simulink model "mech_fceng"  (Simulink 6.0)
settings: Solver=ode45  StartTime=0.0  StopTime=inf  RelTol=1e-3  AbsTol=1e-4
PreLoadFcn:
  | mech_fceng_init;load mech_fceng_images;
InitFcn:
  | mech_slider_open(gcs);
values from neighbouring files (symbols this model uses):
  Cv = 2000    [mech_transmission_data.mat]
  G = 9.81    [mech_motorcycle_data.m]
  m = 161    [mech_transmission_data.mat]
  N = 270    [mech_transmission_data.mat]
  R = 1    [clutchparam.mat]    (also in mech_toroid_setup.m = 10; mech_transmission_data.mat = 5)
undefined symbols (not defined in the file or in its folder): AirRo, Pa, Q, Ta, Vo, Vtdc
libraries: mblibv1 x47, simulink x3, simulink_extras x1
(part 1 of 2)
settings Model: Creator=arnav  LastModifiedBy=batserve  ExtModeAutoUpdateStatusClock=off  ProdHWDeviceType=Specified
settings DataIOCC: SignalLoggingName=sigsOut
settings OptimizationCC: BooleanDataType=off
settings DebuggingCC: CheckExecutionContextPreStartOutputMsg=on  CheckExecutionContextRuntimeOutputMsg=on  SolverPrmCheckMsg=none  UnconnectedInputMsg=none  UnconnectedOutputMsg=none  UnconnectedLineMsg=none
settings HardwareCC: ProdHWDeviceType=Specified
settings SimMechanicsCC: WarnOnRedundantConstraints=off

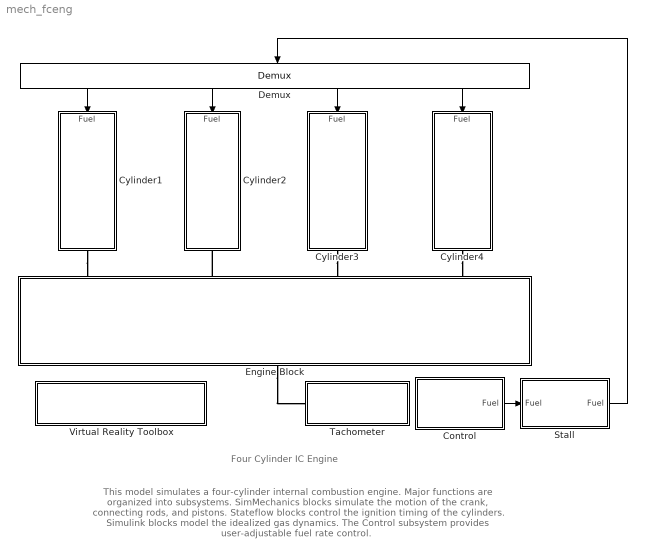
== system mech_fceng ==
  note: This model simulates a four-cylinder internal combustion engine. Major functions are organized into subsystems.
      | SimMechanics blocks simulate the motion of the crank, connecting rods, and pistons. Stateflow blocks
      | control the ignition timing of the cylinders. Simulink blocks model the idealized gas dynamics. The Control
      | subsystem provides user-adjustable fuel rate control.
  note: Four Cylinder IC Engine
  Control : Subsystem  Tag=OpenMeAtStartUp
  Cylinder1 : Subsystem  Orientation=down
      mask Display: image(crodassm);
  Cylinder2 : Subsystem  Orientation=down
      mask Display: image(crodassmb);
  Cylinder3 : Subsystem  Orientation=down
      mask Display: image(crodassmb);
  Cylinder4 : Subsystem  Orientation=down
      mask Display: image(crodassm);
  Demux : Demux  Orientation=down
  Engine Block : Subsystem  Orientation=up
      mask Display: image(crank);
  Stall : Subsystem
  Tachometer : Subsystem
  Virtual Reality Toolbox : Subsystem
      settings: OpenFcn=mech_OpenVrWorld(gcs,'mech_fceng_vrlib')
      mask Type: Double-click open
      mask Display: disp(sprintf('Double-click to open\nVirtual Reality Toolbox viewer'))
  wires:
  Demux/1 -> Cylinder1/1(Fuel)
  Demux/2 -> Cylinder2/1(Fuel)
  Demux/3 -> Cylinder3/1(Fuel)
  Demux/4 -> Cylinder4/1(Fuel)
  Control/1(Fuel) -> Stall/1("Fuel ")
  Stall/1(Fuel) -> Demux/1
  connections:
  Cylinder1/RConn1 -- Engine Block/RConn1
  Cylinder4/RConn1 -- Engine Block/RConn4
  Engine Block/LConn1 -- Tachometer/LConn1
  Cylinder3/RConn1 -- Engine Block/RConn3
  Engine Block/RConn2 -- Cylinder2/RConn1

== system mech_fceng/Control ==
  Constant : Constant
  Cylinder1 : simulink/Signal Routing/Manual Switch  Orientation=down  sw=0  action=0
  Cylinder4 : simulink/Signal Routing/Manual Switch  Orientation=down  sw=0  action=0
  Fuel Control : simulink/Math Operations/Slider Gain  Tag="674   438   332   100"  low=0  gain=2  high=4
  OFF : Constant  Orientation=up  Value=0
  ON : Constant  Orientation=up  Value=-1
  Fuel : Outport
  tag scope: Cylinder1=global, Cylinder2=global
  wires:
  Cylinder1/1 -> [Cylinder1]
  Constant/1 -> Fuel Control/1
  Fuel Control/1 -> Fuel/1
  OFF/1 -> Cylinder1/1, Cylinder4/1
  ON/1 -> Cylinder4/2, Cylinder1/2
  Cylinder4/1 -> [Cylinder2]

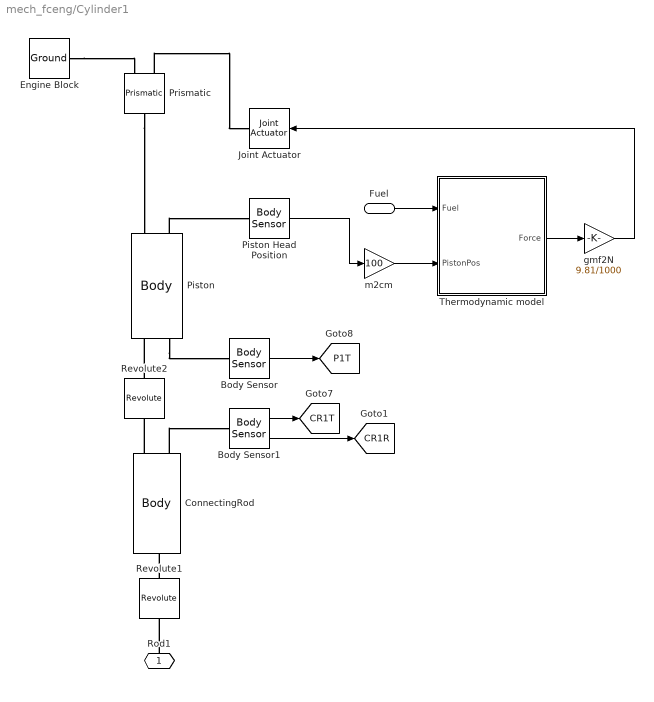
== system mech_fceng/Cylinder1 ==
  Fuel : Inport  Port=1  LatchInput=off
  Body Sensor : mblibv1/Sensors &  Actuators/Body Sensor  Opaque=on  PhysicalDomain=Mechanical  PortType=blob  Muxed=on  Pose=off  Angle=on  AngleUnits=deg  ArcVelocity=off  ArcVelocityUnits=deg/s  ArcAcceleration=off  ArcAccelerationUnits=deg/s^2  CoordPosition=on  CoordPositionUnits=m  Velocity=off  VelocityUnits=m/s  Acceleration=off  AccelerationUnits=m/s^2  Quaternion=on  QuaternionDT=off  QuaternionDDT=off  QuaternionUnits=off  OutputVector=[1]  ActiveIO=on  Width=3  DialogClass=MechanicalSensorBlock  ReferenceFrame=Absolute (World)
  Body Sensor1 : mblibv1/Sensors &  Actuators/Body Sensor  Opaque=on  PhysicalDomain=Mechanical  PortType=blob  Muxed=off  Pose=on  Angle=on  AngleUnits=deg  ArcVelocity=off  ArcVelocityUnits=deg/s  ArcAcceleration=off  ArcAccelerationUnits=deg/s^2  CoordPosition=on  CoordPositionUnits=m  Velocity=off  VelocityUnits=m/s  Acceleration=off  AccelerationUnits=m/s^2  Quaternion=on  QuaternionDT=off  QuaternionDDT=off  QuaternionUnits=off  OutputVector=[ 3 9 ]  ActiveIO=on  Width=12  DialogClass=MechanicalSensorBlock  ReferenceFrame=Absolute (World)
  ConnectingRod : mblibv1/Bodies/Body  Orientation=up  PhysicalDomain=mechanical  SubClassName=Unknown  LeftPortType=workingframe  RightPortType=workingframe  LConnTagsString=CS1  RConnTagsString=CS2|CS3  DialogClass=MechanicalBodyBlock  Mass=676.73  MassUnits=g  InertiaUnits=kg*m^2  Inertia=[37007.64 0 -0.01;0 2936.99 7181.27;-0.01 7181.27 34460.53]*1E-7  Shape=Cylinder  ShapeDims=[1 1]  ShapeUnits=m  ShapeUse=false  Density=1  DensityUnits=kg/m^3  DensityUse=false  CG=Left$CG$[-18 11.35 -2.70]$WORLD$WORLD$cm$[0 0 0]$Euler X-Y-Z$deg$WORLD$false  WorkingFrames=Left$CS1$[-18 4.24 -4.24]$WORLD$WORLD$cm$[0 0 0]$Euler X-Y-Z$deg$WORLD$true#Right$CS2$[-18 23.79 0]$WORLD$WORLD$cm$[0 0 0]$Euler X-Y-Z$deg$WORLD$true#Right$CS3$[-18 4.24 -4.24]$WORLD$WORLD$cm$[0 0 0]$Euler X-Y-Z$deg$WORLD$true
  Engine Block : mblibv1/Bodies/Ground  Opaque=on  LeftPortType=env  RightPortType=workingframe  PhysicalDomain=Mechanical  DialogClass=GroundBlock  CoordPosition=[-13.23 23.79 0]  CoordPositionUnits=cm  StateVectorMgrId=-1  MachineId=[0 0]  ShowEnvPort=off
  Joint Actuator : mblibv1/Sensors &  Actuators/Joint Actuator  Orientation=left  Opaque=on  PhysicalDomain=Mechanical  PortType=blob  ActuationStyle=Force  AngleUnits=deg  ArcVelocityUnits=deg/s  ArcAccelerationUnits=deg/s^2  CoordPositionUnits=m  VelocityUnits=m/s  AccelerationUnits=m/s^2  ForceUnits=N  TorqueUnits=N-m  ActiveIO=on  Width=1  DialogClass=MechanicalActuatorBlock  Primitive=P1  ReferenceFrame=Absolute (INERTIAL)
  Piston : mblibv1/Bodies/Body  Orientation=up  PhysicalDomain=mechanical  SubClassName=Unknown  LeftPortType=workingframe  RightPortType=workingframe  LConnTagsString=CS1|CS3  RConnTagsString=CS2|CS4  DialogClass=MechanicalBodyBlock  Mass=3490.25  MassUnits=g  InertiaUnits=kg*m^2  Inertia=[39798.30 0.06 -0.01;0.06 49173.25 -0.04;-0.01 -0.04 39108.48]*1E-7  Shape=Cylinder  ShapeDims=[1 1]  ShapeUnits=m  ShapeUse=false  Density=1  DensityUnits=kg/m^3  DensityUse=false  CG=Left$CG$[-18 24.51 0]$WORLD$WORLD$cm$[0 0 0]$Euler X-Y-Z$deg$WORLD$false  WorkingFrames=Left$CS1$[-18 23.79 0]$WORLD$WORLD$cm$[0 0 0]$Euler X-Y-Z$deg$WORLD$true#Right$CS2$[-13.23 23.79 0]$WORLD$WORLD$cm$[0 0 0]$Euler X-Y-Z$deg$WORLD$true#Left$CS3$[-18 23.79 0]$WORLD$WORLD$cm$[0 0 0]$Euler X-Y-Z$deg$WORLD$true#Right$CS4$[-18 23.79+4 0]$WORLD$WORLD$cm$[0 0 0]$Euler X-Y-Z$deg$WORLD$true
  Piston Head Position : mblibv1/Sensors &  Actuators/Body Sensor  Opaque=on  PhysicalDomain=Mechanical  PortType=blob  Muxed=on  Pose=off  Angle=on  AngleUnits=deg  ArcVelocity=off  ArcVelocityUnits=deg/s  ArcAcceleration=off  ArcAccelerationUnits=deg/s^2  CoordPosition=on  CoordPositionUnits=m  Velocity=off  VelocityUnits=m/s  Acceleration=off  AccelerationUnits=m/s^2  Quaternion=on  QuaternionDT=off  QuaternionDDT=off  QuaternionUnits=off  OutputVector=[1]  ActiveIO=on  Width=3  DialogClass=MechanicalSensorBlock  ReferenceFrame=Absolute (World)
  Prismatic : mblibv1/Joints/Prismatic  Orientation=down  PhysicalDomain=mechanical  SubClassName=Unknown  LeftPortType=blob  RightPortType=blob  LConnTagsString=__newl0|SA1  RConnTagsString=__newr0  NumSAPorts=1  CutJoint=off  MarkAsCut=off  Primitives=prismatic  PrimitiveProps=P1$WORLD$[0 1 0]$prismatic  DialogClass=JointBlock
  Revolute1 : mblibv1/Joints/Revolute  Orientation=up  PhysicalDomain=mechanical  SubClassName=Unknown  LeftPortType=blob  RightPortType=blob  LConnTagsString=__newl0  RConnTagsString=__newr0  NumSAPorts=0  CutJoint=off  MarkAsCut=off  Primitives=revolute  PrimitiveProps=R1$WORLD$[1 0 0]$revolute  DialogClass=JointBlock
  Revolute2 : mblibv1/Joints/Revolute  Orientation=up  PhysicalDomain=mechanical  SubClassName=Unknown  LeftPortType=blob  RightPortType=blob  LConnTagsString=__newl0  RConnTagsString=__newr0  NumSAPorts=0  CutJoint=on  MarkAsCut=off  Primitives=revolute  PrimitiveProps=R1$WORLD$[1 0 0]$revolute  DialogClass=JointBlock
  Thermodynamic model : Subsystem
  gmf2N : Gain  Gain=9.81/1000  SaturateOnIntegerOverflow=on
  m2cm : Gain  Gain=100  SaturateOnIntegerOverflow=on
  Rod1 : PMIOPort  Orientation=up  Port=1  Side=Right
  tag scope: CR1R=global, CR1T=global, P1T=global
  wires:
  Body Sensor1/2 -> [CR1R]
  Body Sensor1/1 -> [CR1T]
  Body Sensor/1 -> [P1T]
  gmf2N/1 -> Joint Actuator/1
  Fuel/1 -> Thermodynamic model/1(Fuel)
  Piston Head Position/1 -> m2cm/1
  Thermodynamic model/1(Force) -> gmf2N/1
  m2cm/1 -> Thermodynamic model/2(PistonPos)
  connections:
  Prismatic/LConn2 -- Joint Actuator/RConn1
  Prismatic/RConn1 -- Piston/RConn1
  Engine Block/RConn1 -- Prismatic/LConn1
  ConnectingRod/RConn2 -- Body Sensor1/LConn1
  Piston/LConn2 -- Body Sensor/LConn1
  Piston/RConn2 -- Piston Head Position/LConn1
  Rod1/RConn1 -- Revolute1/LConn1
  Revolute2/RConn1 -- Piston/LConn1
  ConnectingRod/RConn1 -- Revolute2/LConn1
  Revolute1/RConn1 -- ConnectingRod/LConn1

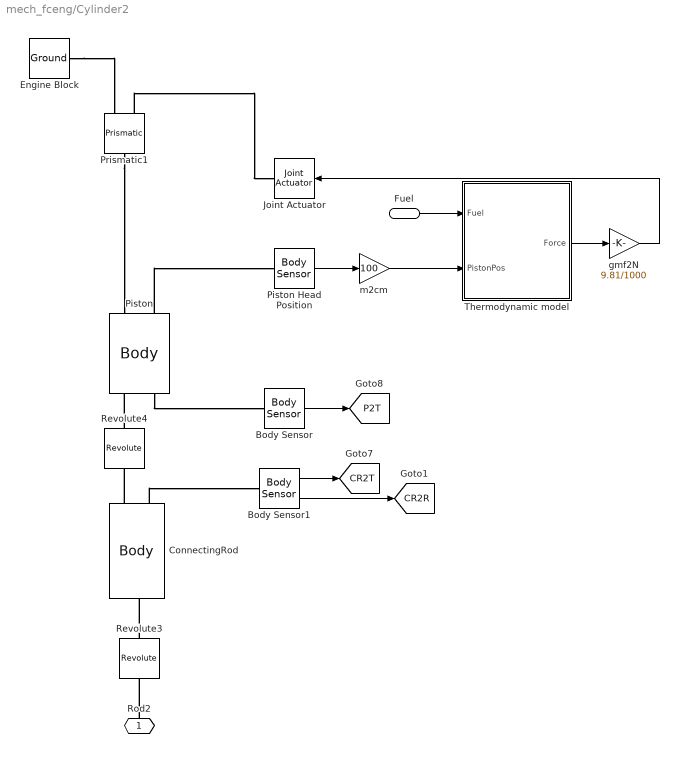
== system mech_fceng/Cylinder2 ==
  Fuel : Inport  Port=1  LatchInput=off
  Body Sensor : mblibv1/Sensors &  Actuators/Body Sensor  Opaque=on  PhysicalDomain=Mechanical  PortType=blob  Muxed=on  Pose=off  Angle=on  AngleUnits=deg  ArcVelocity=off  ArcVelocityUnits=deg/s  ArcAcceleration=off  ArcAccelerationUnits=deg/s^2  CoordPosition=on  CoordPositionUnits=m  Velocity=off  VelocityUnits=m/s  Acceleration=off  AccelerationUnits=m/s^2  Quaternion=on  QuaternionDT=off  QuaternionDDT=off  QuaternionUnits=off  OutputVector=[1]  ActiveIO=on  Width=3  DialogClass=MechanicalSensorBlock  ReferenceFrame=Absolute (World)
  Body Sensor1 : mblibv1/Sensors &  Actuators/Body Sensor  Opaque=on  PhysicalDomain=Mechanical  PortType=blob  Muxed=off  Pose=on  Angle=on  AngleUnits=deg  ArcVelocity=off  ArcVelocityUnits=deg/s  ArcAcceleration=off  ArcAccelerationUnits=deg/s^2  CoordPosition=on  CoordPositionUnits=m  Velocity=off  VelocityUnits=m/s  Acceleration=off  AccelerationUnits=m/s^2  Quaternion=on  QuaternionDT=off  QuaternionDDT=off  QuaternionUnits=off  OutputVector=[ 3 9 ]  ActiveIO=on  Width=12  DialogClass=MechanicalSensorBlock  ReferenceFrame=Absolute (World)
  ConnectingRod : mblibv1/Bodies/Body  Orientation=up  PhysicalDomain=mechanical  SubClassName=Unknown  LeftPortType=workingframe  RightPortType=workingframe  LConnTagsString=CS1  RConnTagsString=CS2|CS3  DialogClass=MechanicalBodyBlock  Mass=676.73  MassUnits=g  InertiaUnits=kg*m^2  Inertia=[37007.64 0 -0.01;0 2936.99 7181.27;-0.01 7181.27 34460.53]*1E-7  Shape=Cylinder  ShapeDims=[1 1]  ShapeUnits=m  ShapeUse=false  Density=1  DensityUnits=kg/m^3  DensityUse=false  CG=Left$CG$[-6 2.87 2.70]$WORLD$WORLD$cm$[0 0 0]$Euler X-Y-Z$deg$WORLD$false  WorkingFrames=Left$CS1$[-6 -4.24 4.24]$WORLD$WORLD$cm$[0 0 0]$Euler X-Y-Z$deg$WORLD$true#Right$CS2$[-6 15.30 0]$WORLD$WORLD$cm$[0 0 0]$Euler X-Y-Z$deg$WORLD$true#Right$CS3$[-6 -4.24 4.24]$WORLD$WORLD$cm$[0 0 0]$Euler X-Y-Z$deg$WORLD$true
  Engine Block : mblibv1/Bodies/Ground  Opaque=on  LeftPortType=env  RightPortType=workingframe  PhysicalDomain=Mechanical  DialogClass=GroundBlock  CoordPosition=[-1 15.30 0]  CoordPositionUnits=cm  StateVectorMgrId=-1  MachineId=[0 0]  ShowEnvPort=off
  Joint Actuator : mblibv1/Sensors &  Actuators/Joint Actuator  Orientation=left  Opaque=on  PhysicalDomain=Mechanical  PortType=blob  ActuationStyle=Force  AngleUnits=deg  ArcVelocityUnits=deg/s  ArcAccelerationUnits=deg/s^2  CoordPositionUnits=m  VelocityUnits=m/s  AccelerationUnits=m/s^2  ForceUnits=N  TorqueUnits=N-m  ActiveIO=on  Width=1  DialogClass=MechanicalActuatorBlock  Primitive=P1  ReferenceFrame=Absolute (INERTIAL)
  Piston : mblibv1/Bodies/Body  Orientation=up  PhysicalDomain=mechanical  SubClassName=Unknown  LeftPortType=workingframe  RightPortType=workingframe  LConnTagsString=CS1|CS3  RConnTagsString=CS2|CS4  DialogClass=MechanicalBodyBlock  Mass=3490.25  MassUnits=g  InertiaUnits=kg*m^2  Inertia=[39798.30 0.06 -0.01;0.06 49173.25 -0.04;-0.01 -0.04 39108.48]*1E-7  Shape=Cylinder  ShapeDims=[1 1]  ShapeUnits=m  ShapeUse=false  Density=1  DensityUnits=kg/m^3  DensityUse=false  CG=Left$CG$[-6 16.02 0]$WORLD$WORLD$cm$[0 0 0]$Euler X-Y-Z$deg$WORLD$false  WorkingFrames=Left$CS1$[-6 15.30 0]$WORLD$WORLD$cm$[0 0 0]$Euler X-Y-Z$deg$WORLD$true#Right$CS2$[-1 15.30 0]$WORLD$WORLD$cm$[0 0 0]$Euler X-Y-Z$deg$WORLD$true#Left$CS3$[-6 15.30 0]$WORLD$WORLD$cm$[0 0 0]$Euler X-Y-Z$deg$WORLD$true#Right$CS4$[-6 19.30 0]$WORLD$WORLD$cm$[0 0 0]$Euler X-Y-Z$deg$WORLD$true
  Piston Head Position : mblibv1/Sensors &  Actuators/Body Sensor  Opaque=on  PhysicalDomain=Mechanical  PortType=blob  Muxed=on  Pose=off  Angle=on  AngleUnits=deg  ArcVelocity=off  ArcVelocityUnits=deg/s  ArcAcceleration=off  ArcAccelerationUnits=deg/s^2  CoordPosition=on  CoordPositionUnits=m  Velocity=off  VelocityUnits=m/s  Acceleration=off  AccelerationUnits=m/s^2  Quaternion=on  QuaternionDT=off  QuaternionDDT=off  QuaternionUnits=off  OutputVector=[1]  ActiveIO=on  Width=3  DialogClass=MechanicalSensorBlock  ReferenceFrame=Absolute (World)
  Prismatic1 : mblibv1/Joints/Prismatic  Orientation=down  PhysicalDomain=mechanical  SubClassName=Unknown  LeftPortType=blob  RightPortType=blob  LConnTagsString=__newl0|SA1  RConnTagsString=__newr0  NumSAPorts=1  CutJoint=off  MarkAsCut=off  Primitives=prismatic  PrimitiveProps=P1$WORLD$[0 1 0]$prismatic  DialogClass=JointBlock
  Revolute3 : mblibv1/Joints/Revolute  Orientation=up  PhysicalDomain=mechanical  SubClassName=Unknown  LeftPortType=blob  RightPortType=blob  LConnTagsString=__newl0  RConnTagsString=__newr0  NumSAPorts=0  CutJoint=off  MarkAsCut=off  Primitives=revolute  PrimitiveProps=R1$WORLD$[1 0 0]$revolute  DialogClass=JointBlock
  Revolute4 : mblibv1/Joints/Revolute  Orientation=up  PhysicalDomain=mechanical  SubClassName=Unknown  LeftPortType=blob  RightPortType=blob  LConnTagsString=__newl0  RConnTagsString=__newr0  NumSAPorts=0  CutJoint=on  MarkAsCut=off  Primitives=revolute  PrimitiveProps=R1$WORLD$[1 0 0]$revolute  DialogClass=JointBlock
  Thermodynamic model : Subsystem
  gmf2N : Gain  Gain=9.81/1000  SaturateOnIntegerOverflow=on
  m2cm : Gain  Gain=100  SaturateOnIntegerOverflow=on
  Rod2 : PMIOPort  Orientation=up  Port=1  Side=Right
  tag scope: CR2R=global, CR2T=global, P2T=global
  wires:
  Body Sensor1/2 -> [CR2R]
  Body Sensor/1 -> [P2T]
  Body Sensor1/1 -> [CR2T]
  gmf2N/1 -> Joint Actuator/1
  Fuel/1 -> Thermodynamic model/1(Fuel)
  Piston Head Position/1 -> m2cm/1
  Thermodynamic model/1(Force) -> gmf2N/1
  m2cm/1 -> Thermodynamic model/2(PistonPos)
  connections:
  Prismatic1/LConn2 -- Joint Actuator/RConn1
  Prismatic1/RConn1 -- Piston/RConn1
  Engine Block/RConn1 -- Prismatic1/LConn1
  ConnectingRod/RConn2 -- Body Sensor1/LConn1
  Piston/LConn2 -- Body Sensor/LConn1
  Piston/RConn2 -- Piston Head Position/LConn1
  Revolute3/RConn1 -- ConnectingRod/LConn1
  ConnectingRod/RConn1 -- Revolute4/LConn1
  Revolute4/RConn1 -- Piston/LConn1
  Rod2/RConn1 -- Revolute3/LConn1

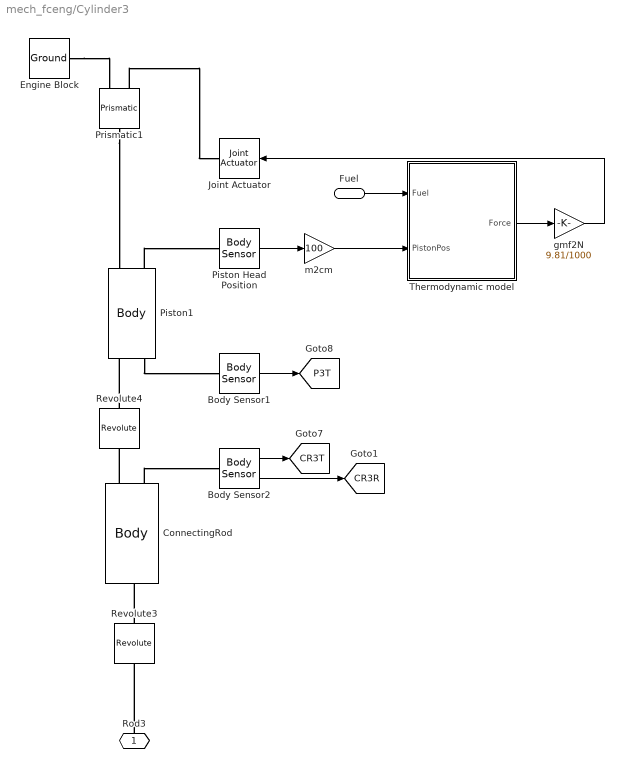
== system mech_fceng/Cylinder3 ==
  Fuel : Inport  Port=1  LatchInput=off
  Body Sensor1 : mblibv1/Sensors &  Actuators/Body Sensor  Opaque=on  PhysicalDomain=Mechanical  PortType=blob  Muxed=on  Pose=off  Angle=on  AngleUnits=deg  ArcVelocity=off  ArcVelocityUnits=deg/s  ArcAcceleration=off  ArcAccelerationUnits=deg/s^2  CoordPosition=on  CoordPositionUnits=m  Velocity=off  VelocityUnits=m/s  Acceleration=off  AccelerationUnits=m/s^2  Quaternion=on  QuaternionDT=off  QuaternionDDT=off  QuaternionUnits=off  OutputVector=[1]  ActiveIO=on  Width=3  DialogClass=MechanicalSensorBlock  ReferenceFrame=Absolute (World)
  Body Sensor2 : mblibv1/Sensors &  Actuators/Body Sensor  Opaque=on  PhysicalDomain=Mechanical  PortType=blob  Muxed=off  Pose=on  Angle=on  AngleUnits=deg  ArcVelocity=off  ArcVelocityUnits=deg/s  ArcAcceleration=off  ArcAccelerationUnits=deg/s^2  CoordPosition=on  CoordPositionUnits=m  Velocity=off  VelocityUnits=m/s  Acceleration=off  AccelerationUnits=m/s^2  Quaternion=on  QuaternionDT=off  QuaternionDDT=off  QuaternionUnits=off  OutputVector=[ 3 9 ]  ActiveIO=on  Width=12  DialogClass=MechanicalSensorBlock  ReferenceFrame=Absolute (World)
  ConnectingRod : mblibv1/Bodies/Body  Orientation=up  PhysicalDomain=mechanical  SubClassName=Unknown  LeftPortType=workingframe  RightPortType=workingframe  LConnTagsString=CS1  RConnTagsString=CS2|CS3  DialogClass=MechanicalBodyBlock  Mass=676.73  MassUnits=g  InertiaUnits=kg*m^2  Inertia=[37007.64 0 -0.01;0 2936.99 7181.27;-0.01 7181.27 34460.53]*1E-7  Shape=Cylinder  ShapeDims=[1 1]  ShapeUnits=m  ShapeUse=false  Density=1  DensityUnits=kg/m^3  DensityUse=false  CG=Left$CG$[6 2.87 2.70]$WORLD$WORLD$cm$[0 0 0]$Euler X-Y-Z$deg$WORLD$false  WorkingFrames=Left$CS1$[6 -4.24 4.24]$WORLD$WORLD$cm$[0 0 0]$Euler X-Y-Z$deg$WORLD$true#Right$CS2$[6 15.30 0]$WORLD$WORLD$cm$[0 0 0]$Euler X-Y-Z$deg$WORLD$true#Right$CS3$[6 -4.24 4.24]$WORLD$WORLD$cm$[0 0 0]$Euler X-Y-Z$deg$WORLD$true
  Engine Block : mblibv1/Bodies/Ground  Opaque=on  LeftPortType=env  RightPortType=workingframe  PhysicalDomain=Mechanical  DialogClass=GroundBlock  CoordPosition=[11 15.30 0]  CoordPositionUnits=cm  StateVectorMgrId=-1  MachineId=[0 0]  ShowEnvPort=off
  Joint Actuator : mblibv1/Sensors &  Actuators/Joint Actuator  Orientation=left  Opaque=on  PhysicalDomain=Mechanical  PortType=blob  ActuationStyle=Force  AngleUnits=deg  ArcVelocityUnits=deg/s  ArcAccelerationUnits=deg/s^2  CoordPositionUnits=m  VelocityUnits=m/s  AccelerationUnits=m/s^2  ForceUnits=N  TorqueUnits=N-m  ActiveIO=on  Width=1  DialogClass=MechanicalActuatorBlock  Primitive=P1  ReferenceFrame=Absolute (INERTIAL)
  Piston Head Position : mblibv1/Sensors &  Actuators/Body Sensor  Opaque=on  PhysicalDomain=Mechanical  PortType=blob  Muxed=on  Pose=off  Angle=on  AngleUnits=deg  ArcVelocity=off  ArcVelocityUnits=deg/s  ArcAcceleration=off  ArcAccelerationUnits=deg/s^2  CoordPosition=on  CoordPositionUnits=m  Velocity=off  VelocityUnits=m/s  Acceleration=off  AccelerationUnits=m/s^2  Quaternion=on  QuaternionDT=off  QuaternionDDT=off  QuaternionUnits=off  OutputVector=[1]  ActiveIO=on  Width=3  DialogClass=MechanicalSensorBlock  ReferenceFrame=Absolute (World)
  Piston1 : mblibv1/Bodies/Body  Orientation=up  PhysicalDomain=mechanical  SubClassName=Unknown  LeftPortType=workingframe  RightPortType=workingframe  LConnTagsString=CS1|CS3  RConnTagsString=CS2|CS4  DialogClass=MechanicalBodyBlock  Mass=3490.25  MassUnits=g  InertiaUnits=kg*m^2  Inertia=[39798.30 0.06 -0.01;0.06 49173.25 -0.04;-0.01 -0.04 39108.48]*1E-7  Shape=Cylinder  ShapeDims=[1 1]  ShapeUnits=m  ShapeUse=false  Density=1  DensityUnits=kg/m^3  DensityUse=false  CG=Left$CG$[6 16.02 0]$WORLD$WORLD$cm$[0 0 0]$Euler X-Y-Z$deg$WORLD$false  WorkingFrames=Left$CS1$[6 15.30 0]$WORLD$WORLD$cm$[0 0 0]$Euler X-Y-Z$deg$WORLD$true#Right$CS2$[11 15.30 0]$WORLD$WORLD$cm$[0 0 0]$Euler X-Y-Z$deg$WORLD$true#Left$CS3$[6 15.30 0]$WORLD$WORLD$cm$[0 0 0]$Euler X-Y-Z$deg$WORLD$true#Right$CS4$[6 15.30+4 0]$WORLD$WORLD$cm$[0 0 0]$Euler X-Y-Z$deg$WORLD$true
  Prismatic1 : mblibv1/Joints/Prismatic  Orientation=down  PhysicalDomain=mechanical  SubClassName=Unknown  LeftPortType=blob  RightPortType=blob  LConnTagsString=__newl0|SA1  RConnTagsString=__newr0  NumSAPorts=1  CutJoint=off  MarkAsCut=off  Primitives=prismatic  PrimitiveProps=P1$WORLD$[0 1 0]$prismatic  DialogClass=JointBlock
  Revolute3 : mblibv1/Joints/Revolute  Orientation=up  PhysicalDomain=mechanical  SubClassName=Unknown  LeftPortType=blob  RightPortType=blob  LConnTagsString=__newl0  RConnTagsString=__newr0  NumSAPorts=0  CutJoint=off  MarkAsCut=off  Primitives=revolute  PrimitiveProps=R1$WORLD$[1 0 0]$revolute  DialogClass=JointBlock
  Revolute4 : mblibv1/Joints/Revolute  Orientation=up  PhysicalDomain=mechanical  SubClassName=Unknown  LeftPortType=blob  RightPortType=blob  LConnTagsString=__newl0  RConnTagsString=__newr0  NumSAPorts=0  CutJoint=on  MarkAsCut=off  Primitives=revolute  PrimitiveProps=R1$WORLD$[1 0 0]$revolute  DialogClass=JointBlock
  Thermodynamic model : Subsystem
  gmf2N : Gain  Gain=9.81/1000  SaturateOnIntegerOverflow=on
  m2cm : Gain  Gain=100  SaturateOnIntegerOverflow=on
  Rod3 : PMIOPort  Orientation=up  Port=1  Side=Right
  tag scope: CR3R=global, CR3T=global, P3T=global
  wires:
  Body Sensor2/2 -> [CR3R]
  Body Sensor2/1 -> [CR3T]
  Body Sensor1/1 -> [P3T]
  gmf2N/1 -> Joint Actuator/1
  Fuel/1 -> Thermodynamic model/1(Fuel)
  Piston Head Position/1 -> m2cm/1
  Thermodynamic model/1(Force) -> gmf2N/1
  m2cm/1 -> Thermodynamic model/2(PistonPos)
  connections:
  Prismatic1/LConn2 -- Joint Actuator/RConn1
  Prismatic1/RConn1 -- Piston1/RConn1
  Engine Block/RConn1 -- Prismatic1/LConn1
  Piston1/LConn2 -- Body Sensor1/LConn1
  ConnectingRod/RConn2 -- Body Sensor2/LConn1
  Rod3/RConn1 -- Revolute3/LConn1
  Revolute4/RConn1 -- Piston1/LConn1
  ConnectingRod/RConn1 -- Revolute4/LConn1
  Revolute3/RConn1 -- ConnectingRod/LConn1
  Piston1/RConn2 -- Piston Head Position/LConn1

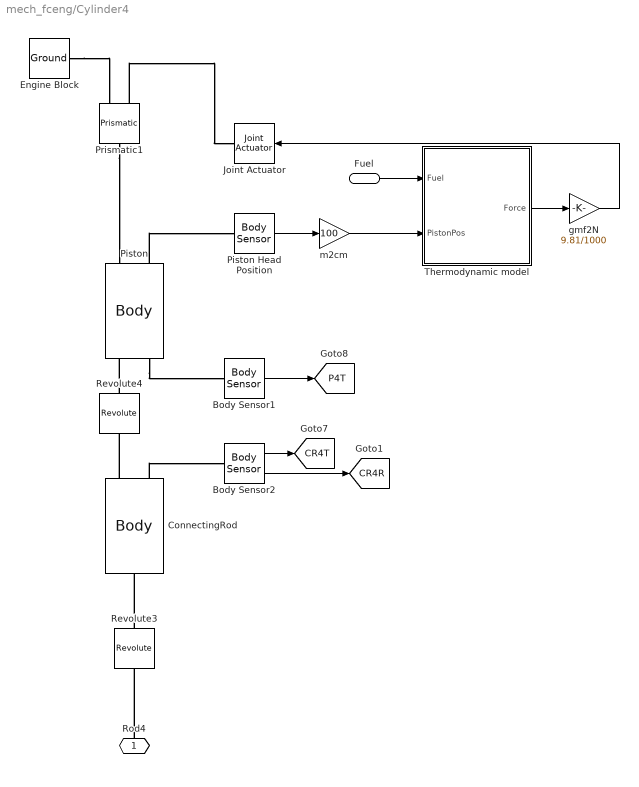
== system mech_fceng/Cylinder4 ==
  Fuel : Inport  Port=1  LatchInput=off
  Body Sensor1 : mblibv1/Sensors &  Actuators/Body Sensor  Opaque=on  PhysicalDomain=Mechanical  PortType=blob  Muxed=on  Pose=off  Angle=on  AngleUnits=deg  ArcVelocity=off  ArcVelocityUnits=deg/s  ArcAcceleration=off  ArcAccelerationUnits=deg/s^2  CoordPosition=on  CoordPositionUnits=m  Velocity=off  VelocityUnits=m/s  Acceleration=off  AccelerationUnits=m/s^2  Quaternion=on  QuaternionDT=off  QuaternionDDT=off  QuaternionUnits=off  OutputVector=[1]  ActiveIO=on  Width=3  DialogClass=MechanicalSensorBlock  ReferenceFrame=Absolute (INERTIAL)
  Body Sensor2 : mblibv1/Sensors &  Actuators/Body Sensor  Opaque=on  PhysicalDomain=Mechanical  PortType=blob  Muxed=off  Pose=on  Angle=on  AngleUnits=deg  ArcVelocity=off  ArcVelocityUnits=deg/s  ArcAcceleration=off  ArcAccelerationUnits=deg/s^2  CoordPosition=on  CoordPositionUnits=m  Velocity=off  VelocityUnits=m/s  Acceleration=off  AccelerationUnits=m/s^2  Quaternion=on  QuaternionDT=off  QuaternionDDT=off  QuaternionUnits=off  OutputVector=[ 3 9 ]  ActiveIO=on  Width=12  DialogClass=MechanicalSensorBlock  ReferenceFrame=Absolute (World)
  ConnectingRod : mblibv1/Bodies/Body  Orientation=up  PhysicalDomain=mechanical  SubClassName=Unknown  LeftPortType=workingframe  RightPortType=workingframe  LConnTagsString=CS1  RConnTagsString=CS2|CS3  DialogClass=MechanicalBodyBlock  Mass=676.73  MassUnits=g  InertiaUnits=kg*m^2  Inertia=[37007.64 0 -0.01;0 2936.99 7181.27;-0.01 7181.27 34460.53]*1E-7  Shape=Cylinder  ShapeDims=[1 1]  ShapeUnits=m  ShapeUse=false  Density=1  DensityUnits=kg/m^3  DensityUse=false  CG=Left$CG$[18 11.35 -2.70]$WORLD$WORLD$cm$[0 0 0]$Euler X-Y-Z$deg$WORLD$false  WorkingFrames=Left$CS1$[18 4.24 -4.24]$WORLD$WORLD$cm$[0 0 0]$Euler X-Y-Z$deg$WORLD$true#Right$CS2$[18 23.79 0]$WORLD$WORLD$cm$[0 0 0]$Euler X-Y-Z$deg$WORLD$true#Right$CS3$[18 4.24 -4.24]$WORLD$WORLD$cm$[0 0 0]$Euler X-Y-Z$deg$WORLD$true
  Engine Block : mblibv1/Bodies/Ground  Opaque=on  LeftPortType=env  RightPortType=workingframe  PhysicalDomain=Mechanical  DialogClass=GroundBlock  CoordPosition=[23 23.79 0]  CoordPositionUnits=cm  StateVectorMgrId=-1  MachineId=[0 0]  ShowEnvPort=off
  Joint Actuator : mblibv1/Sensors &  Actuators/Joint Actuator  Orientation=left  Opaque=on  PhysicalDomain=Mechanical  PortType=blob  ActuationStyle=Force  AngleUnits=deg  ArcVelocityUnits=deg/s  ArcAccelerationUnits=deg/s^2  CoordPositionUnits=m  VelocityUnits=m/s  AccelerationUnits=m/s^2  ForceUnits=N  TorqueUnits=N-m  ActiveIO=on  Width=1  DialogClass=MechanicalActuatorBlock  Primitive=P1  ReferenceFrame=Absolute (INERTIAL)
  Piston : mblibv1/Bodies/Body  Orientation=up  PhysicalDomain=mechanical  SubClassName=Unknown  LeftPortType=workingframe  RightPortType=workingframe  LConnTagsString=CS1|CS3  RConnTagsString=CS2|CS4  DialogClass=MechanicalBodyBlock  Mass=3490.25  MassUnits=g  InertiaUnits=kg*m^2  Inertia=[39798.30 0.06 -0.01;0.06 49173.25 -0.04;-0.01 -0.04 39108.48]*1E-7  Shape=Cylinder  ShapeDims=[1 1]  ShapeUnits=m  ShapeUse=false  Density=1  DensityUnits=kg/m^3  DensityUse=false  CG=Left$CG$[18 24.51 0]$WORLD$WORLD$cm$[0 0 0]$Euler X-Y-Z$deg$WORLD$false  WorkingFrames=Left$CS1$[18 23.79 0]$WORLD$WORLD$cm$[0 0 0]$Euler X-Y-Z$deg$WORLD$true#Right$CS2$[23 23.79 0]$WORLD$WORLD$cm$[0 0 0]$Euler X-Y-Z$deg$WORLD$true#Left$CS3$[18 23.79 0]$WORLD$WORLD$cm$[0 0 0]$Euler X-Y-Z$deg$WORLD$true#Right$CS4$[18 23.79+4 0]$WORLD$WORLD$cm$[0 0 0]$Euler X-Y-Z$deg$WORLD$true
  Piston Head Position : mblibv1/Sensors &  Actuators/Body Sensor  Opaque=on  PhysicalDomain=Mechanical  PortType=blob  Muxed=on  Pose=off  Angle=on  AngleUnits=deg  ArcVelocity=off  ArcVelocityUnits=deg/s  ArcAcceleration=off  ArcAccelerationUnits=deg/s^2  CoordPosition=on  CoordPositionUnits=m  Velocity=off  VelocityUnits=m/s  Acceleration=off  AccelerationUnits=m/s^2  Quaternion=on  QuaternionDT=off  QuaternionDDT=off  QuaternionUnits=off  OutputVector=[1]  ActiveIO=on  Width=3  DialogClass=MechanicalSensorBlock  ReferenceFrame=Absolute (World)
  Prismatic1 : mblibv1/Joints/Prismatic  Orientation=down  PhysicalDomain=mechanical  SubClassName=Unknown  LeftPortType=blob  RightPortType=blob  LConnTagsString=__newl0|SA1  RConnTagsString=__newr0  NumSAPorts=1  CutJoint=off  MarkAsCut=off  Primitives=prismatic  PrimitiveProps=P1$WORLD$[0 1 0]$prismatic  DialogClass=JointBlock
  Revolute3 : mblibv1/Joints/Revolute  Orientation=up  PhysicalDomain=mechanical  SubClassName=Unknown  LeftPortType=blob  RightPortType=blob  LConnTagsString=__newl0  RConnTagsString=__newr0  NumSAPorts=0  CutJoint=off  MarkAsCut=off  Primitives=revolute  PrimitiveProps=R1$WORLD$[1 0 0]$revolute  DialogClass=JointBlock
  Revolute4 : mblibv1/Joints/Revolute  Orientation=up  PhysicalDomain=mechanical  SubClassName=Unknown  LeftPortType=blob  RightPortType=blob  LConnTagsString=__newl0  RConnTagsString=__newr0  NumSAPorts=0  CutJoint=on  MarkAsCut=off  Primitives=revolute  PrimitiveProps=R1$WORLD$[1 0 0]$revolute  DialogClass=JointBlock
  Thermodynamic model : Subsystem
  gmf2N : Gain  Gain=9.81/1000  SaturateOnIntegerOverflow=on
  m2cm : Gain  Gain=100  SaturateOnIntegerOverflow=on
  Rod4 : PMIOPort  Orientation=up  Port=1  Side=Right
  tag scope: CR4R=global, CR4T=global, P4T=global
  wires:
  Body Sensor2/2 -> [CR4R]
  Body Sensor2/1 -> [CR4T]
  Body Sensor1/1 -> [P4T]
  m2cm/1 -> Thermodynamic model/2(PistonPos)
  Thermodynamic model/1(Force) -> gmf2N/1
  Piston Head Position/1 -> m2cm/1
  Fuel/1 -> Thermodynamic model/1(Fuel)
  gmf2N/1 -> Joint Actuator/1
  connections:
  Prismatic1/LConn2 -- Joint Actuator/RConn1
  Prismatic1/RConn1 -- Piston/RConn1
  Engine Block/RConn1 -- Prismatic1/LConn1
  ConnectingRod/RConn2 -- Body Sensor2/LConn1
  Piston/LConn2 -- Body Sensor1/LConn1
  Piston/RConn2 -- Piston Head Position/LConn1
  Rod4/RConn1 -- Revolute3/LConn1
  Revolute3/RConn1 -- ConnectingRod/LConn1
  ConnectingRod/RConn1 -- Revolute4/LConn1
  Revolute4/RConn1 -- Piston/LConn1

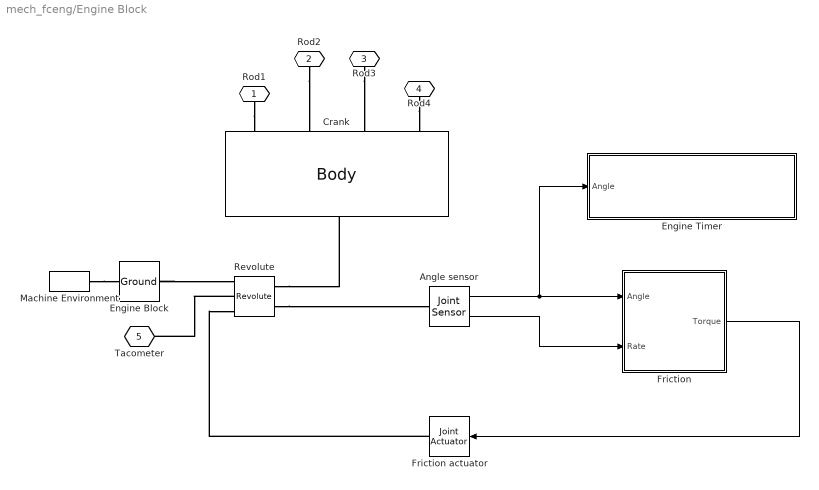
== system mech_fceng/Engine Block ==
  Angle sensor : mblibv1/Sensors &  Actuators/Joint Sensor  Opaque=on  PhysicalDomain=Mechanical  PortType=blob  Muxed=off  Pose=on  Angle=on  AngleUnits=rad  ArcVelocity=on  ArcVelocityUnits=rad/s  ArcAcceleration=off  ArcAccelerationUnits=deg/s^2  CoordPosition=on  CoordPositionUnits=m  Velocity=off  VelocityUnits=m/s  Acceleration=off  AccelerationUnits=m/s^2  Quaternion=on  QuaternionDT=off  QuaternionDDT=off  QuaternionUnits=off  OutputVector=[ 1 1 ]  ActiveIO=on  Width=2  DialogClass=MechanicalSensorBlock  Primitive=R1  Force=off  ForceUnits=N  Torque=off  TorqueUnits=N-m  ReferenceFrame=Absolute (INERTIAL)  ReactionSensedSide=Base  ReactionReferenceFrame=Absolute (World)  ReactionForce=off  ReactionForceUnits=N  ReactionMoment=off  ReactionMomentUnits=N-m
  Crank : mblibv1/Bodies/Body  Orientation=up  PhysicalDomain=mechanical  SubClassName=Unknown  LeftPortType=workingframe  RightPortType=workingframe  LConnTagsString=CS1  RConnTagsString=CS2|CS3|CS4|CS5  DialogClass=MechanicalBodyBlock  Mass=33846.54  MassUnits=g  InertiaUnits=kg*m^2  Inertia=[1159762.55 0 0;0 9246514.71 -187767.86;0 -187767.86 9246514.71]*1E-5  Shape=Cylinder  ShapeDims=[1 1]  ShapeUnits=m  ShapeUse=false  Density=1  DensityUnits=kg/m^3  DensityUse=false  CG=Left$CG$[4.45 0 0]$WORLD$WORLD$cm$[0 0 0]$Euler X-Y-Z$deg$WORLD$false  WorkingFrames=Left$CS1$[0 0 0]$WORLD$WORLD$cm$[0 0 0]$Euler X-Y-Z$deg$WORLD$true#Right$CS2$[-18 4.24 -4.24]$WORLD$WORLD$cm$[0 0 0]$Euler X-Y-Z$deg$WORLD$true#Right$CS3$[-6 -4.24 4.24]$WORLD$WORLD$cm$[0 0 0]$Euler X-Y-Z$deg$WORLD$true#Right$CS4$[6 -4.24 4.24]$WORLD$WORLD$cm$[0 0 0]$Euler X-Y-Z$deg$WORLD$true#Right$CS5$[18 4.24 -4.24]$WORLD$WORLD$cm$[0 0 0]$Euler X-Y-Z$deg$WORLD$true
  Engine Block : mblibv1/Bodies/Ground  Opaque=on  LeftPortType=env  RightPortType=workingframe  PhysicalDomain=Mechanical  DialogClass=GroundBlock  CoordPosition=[0 0 0]  CoordPositionUnits=cm  StateVectorMgrId=-1  MachineId=[0 0]  ShowEnvPort=on
  Engine Timer : Subsystem
  Friction : Subsystem
  Friction actuator : mblibv1/Sensors &  Actuators/Joint Actuator  Orientation=left  Opaque=on  PhysicalDomain=Mechanical  PortType=blob  ActuationStyle=Force  AngleUnits=deg  ArcVelocityUnits=deg/s  ArcAccelerationUnits=deg/s^2  CoordPositionUnits=m  VelocityUnits=m/s  AccelerationUnits=m/s^2  ForceUnits=N  TorqueUnits=N-m  ActiveIO=on  Width=1  DialogClass=MechanicalActuatorBlock  Primitive=R1  ReferenceFrame=Absolute (INERTIAL)
  Machine Environment : mblibv1/Bodies/Machine Environment  Tag=Factory ground  DialogController=MECH.DialogSource  Opaque=on  PortType=env  PhysicalDomain=Mechanical  DialogTemplateClass=MECH.MachineEnvironment  SyncWhenCopied=off  Gravity=[0 -9.81 0]  GravityUnits=m/s^2  GravityAsSignal=off  Dimensionality=3D Only  AnalysisType=Forward dynamics  LinearAssemblyTolerance=1e-3  LinearAssemblyToleranceUnits=m  AngularAssemblyTolerance=1e-3  AngularAssemblyToleranceUnits=rad  ConstraintSolverType=Stabilizing  ConstraintRelTolerance=1e-4  ConstraintAbsTolerance=1e-4  UseRobustSingularityHandling=off  StatePerturbationType=Fixed  PerturbationSize=1e-5  VisualizeMachine=on
  Revolute : mblibv1/Joints/Revolute  PhysicalDomain=mechanical  SubClassName=Unknown  LeftPortType=blob  RightPortType=blob  LConnTagsString=__newl0|SA1|SA2  RConnTagsString=__newr0|SA1  NumSAPorts=3  CutJoint=off  MarkAsCut=off  Primitives=revolute  PrimitiveProps=R1$WORLD$[1 0 0]$revolute  DialogClass=JointBlock
  Rod1 : PMIOPort  Orientation=down  Port=1  Side=Right
  Rod2 : PMIOPort  Orientation=down  Port=2  Side=Right
  Rod3 : PMIOPort  Orientation=down  Port=3  Side=Right
  Rod4 : PMIOPort  Orientation=down  Port=4  Side=Right
  Tacometer : PMIOPort  Port=5  Side=Left
  wires:
  Angle sensor/2 -> Friction/2(Rate)
  Friction/1(Torque) -> Friction actuator/1
  Angle sensor/1 -> Engine Timer/1(Angle), Friction/1(Angle)
  connections:
  Revolute/LConn2 -- Tacometer/RConn1
  Friction actuator/RConn1 -- Revolute/LConn3
  Revolute/RConn2 -- Angle sensor/LConn1
  Engine Block/RConn1 -- Revolute/LConn1
  Revolute/RConn1 -- Crank/LConn1
  Rod4/RConn1 -- Crank/RConn4
  Rod3/RConn1 -- Crank/RConn3
  Rod2/RConn1 -- Crank/RConn2
  Rod1/RConn1 -- Crank/RConn1
  Machine Environment/RConn1 -- Engine Block/LConn1

== system mech_fceng/Stall ==
  "Fuel " : Inport  Port=1  LatchInput=off
  Gain1 : Gain  Orientation=down  Gain=0.05  SaturateOnIntegerOverflow=on
  Gain2 : Gain  Orientation=down  Gain=-1  SaturateOnIntegerOverflow=on
  Gain3 : Gain  Orientation=down  Gain=-1  SaturateOnIntegerOverflow=on
  Mux : Mux  Orientation=down
  Switch : Switch  Orientation=down  Threshold=0.5  ZeroCross=off  InputSameDT=on
  Switch1 : Switch  Orientation=down  Threshold=0.5  ZeroCross=off  InputSameDT=on
  Fuel : Outport  Orientation=down
  wires:
  "Fuel "/1 -> Gain1/1
  Switch/1 -> Mux/1
  Gain1/1 -> Mux/2, Mux/3, Switch/1, Switch1/1
  Switch1/1 -> Mux/4
  Mux/1 -> Fuel/1
  Gain2/1 -> Switch/2
  Gain3/1 -> Switch1/2
  [Cylinder1] -> Gain2/1
  [Cylinder2] -> Gain3/1

== system mech_fceng/Tachometer ==
  note: RPM
  Constant : Constant  Value=0
  Engine RPM : Scope
      settings: Tag=OpenMeAtStartUp  YMin=0  YMax=900  SaveName=ScopeData2
  Gain1 : Gain  Orientation=left  Gain=60/(2*pi)  SaturateOnIntegerOverflow=on
  Joint Sensor : mblibv1/Sensors &  Actuators/Joint Sensor  Orientation=left  Opaque=on  PhysicalDomain=Mechanical  PortType=blob  Muxed=on  Pose=off  Angle=off  AngleUnits=deg  ArcVelocity=on  ArcVelocityUnits=rad/s  ArcAcceleration=off  ArcAccelerationUnits=deg/s^2  CoordPosition=on  CoordPositionUnits=m  Velocity=off  VelocityUnits=m/s  Acceleration=off  AccelerationUnits=m/s^2  Quaternion=on  QuaternionDT=off  QuaternionDDT=off  QuaternionUnits=off  OutputVector=[ 1 ]  ActiveIO=on  Width=1  DialogClass=MechanicalSensorBlock  Primitive=R1  Force=off  ForceUnits=N  Torque=off  TorqueUnits=N-m  ReferenceFrame=Absolute (INERTIAL)  ReactionSensedSide=Base  ReactionReferenceFrame=Absolute (World)  ReactionForce=off  ReactionForceUnits=N  ReactionMoment=off  ReactionMomentUnits=N-m
  Relational Operator : RelationalOperator  Operator=<  ZeroCross=off  InputSameDT=on
  Stop Simulation : Stop
  Transfer Fcn : TransferFcn  Orientation=left  Numerator=[15]  Denominator=[1 15]
  Rate : PMIOPort  Tag=PMCPort  Orientation=left  Port=1  Side=Left
  wires:
  Gain1/1 -> Relational Operator/1, Transfer Fcn/1
  Constant/1 -> Relational Operator/2
  Joint Sensor/1 -> Gain1/1
  Relational Operator/1 -> Stop Simulation/1
  Transfer Fcn/1 -> Engine RPM/1  "RPM"
  connections:
  Rate/RConn1 -- Joint Sensor/LConn1

== system mech_fceng/Virtual Reality Toolbox ==

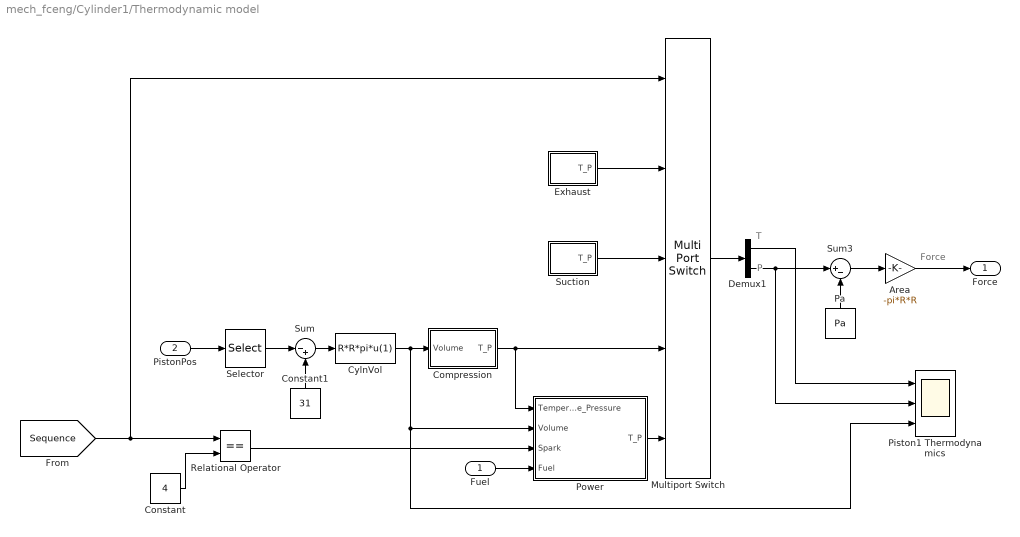
== system mech_fceng/Cylinder1/Thermodynamic model ==
  note: Force
  note: P
  note: T
  Fuel : Inport  Port=1  LatchInput=off
  PistonPos : Inport  Port=2  LatchInput=off
  Area : Gain  Gain=-pi*R*R  SaturateOnIntegerOverflow=on
  Compression : Subsystem
  Constant : Constant  Value=4
  Constant1 : Constant  Orientation=up  Value=31
  CylnVol : Fcn  Expr=R*R*pi*u(1)
  Demux1 : Demux  Outputs=2
  Exhaust : Subsystem  TreatAsAtomicUnit=on
  Multiport Switch : MultiPortSwitch  InputSameDT=on
  Pa : Constant  Orientation=up  Value=Pa
  Piston1 Thermodynamics : Scope  NumInputPorts=3
      settings: YMin=25~0~50  YMax=425~240000~1050
  Power : Subsystem
  Relational Operator : RelationalOperator  Operator===  ZeroCross=off  InputSameDT=on
  Selector : Selector  Elements=2  InputPortWidth=3
  Suction : Subsystem  TreatAsAtomicUnit=on
  Sum : Sum  Inputs=|-+  SaturateOnIntegerOverflow=on  InputSameDT=on
  Sum3 : Sum  Inputs=|+-  SaturateOnIntegerOverflow=on  InputSameDT=on
  Force : Outport
  wires:
  PistonPos/1 -> Selector/1
  Selector/1 -> Sum/1
  [Sequence] -> Multiport Switch/1, Relational Operator/1
  Relational Operator/1 -> Power/3(Spark)
  Area/1 -> Force/1
  Sum/1 -> CylnVol/1
  Constant/1 -> Relational Operator/2
  Demux1/1 -> Piston1 Thermodynamics/1
  Compression/1(T_P) -> Multiport Switch/4, Power/1(Temperature_Pressure)
  CylnVol/1 -> Piston1 Thermodynamics/3, Power/2(Volume), Compression/1(Volume)
  Constant1/1 -> Sum/2
  Fuel/1 -> Power/4(Fuel)
  Power/1(T_P) -> Multiport Switch/5
  Demux1/2 -> Piston1 Thermodynamics/2, Sum3/1
  Sum3/1 -> Area/1
  Pa/1 -> Sum3/2
  Multiport Switch/1 -> Demux1/1
  Exhaust/1(T_P) -> Multiport Switch/2
  Suction/1(T_P) -> Multiport Switch/3

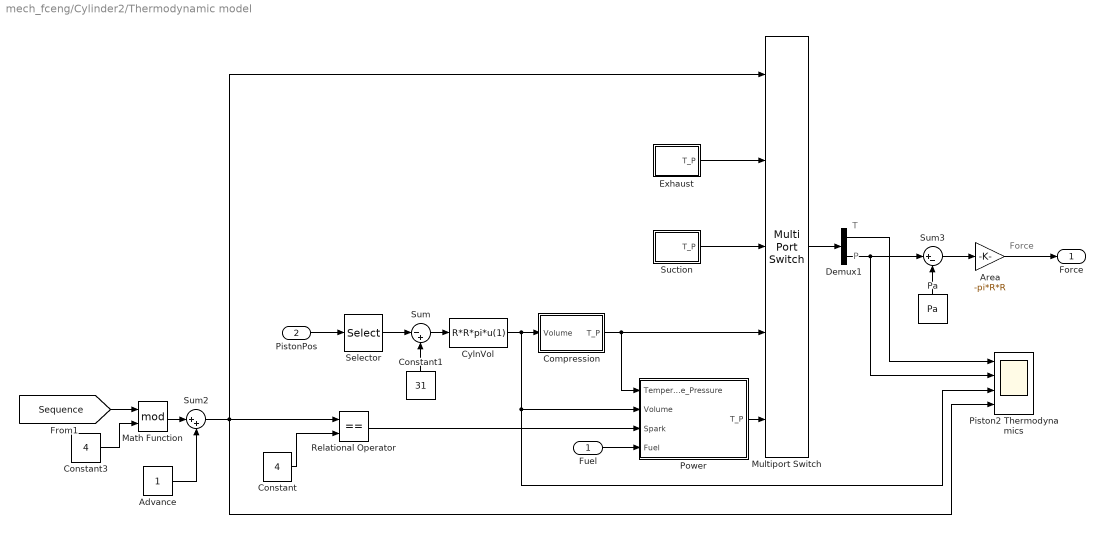
== system mech_fceng/Cylinder2/Thermodynamic model ==
  note: Force
  note: P
  note: T
  Fuel : Inport  Port=1  LatchInput=off
  PistonPos : Inport  Port=2  LatchInput=off
  Advance : Constant
  Area : Gain  Gain=-pi*R*R  SaturateOnIntegerOverflow=on
  Compression : Subsystem
  Constant : Constant  Value=4
  Constant1 : Constant  Orientation=up  Value=31
  Constant3 : Constant  Value=4
  CylnVol : Fcn  Expr=R*R*pi*u(1)
  Demux1 : Demux  Outputs=2
  Exhaust : Subsystem  TreatAsAtomicUnit=on
  Math Function : Math  Operator=mod  SaturateOnIntegerOverflow=on
  Multiport Switch : MultiPortSwitch  InputSameDT=on
  Pa : Constant  Orientation=up  Value=Pa
  Piston2 Thermodynamics : Scope  NumInputPorts=4
      settings: YMin=20~0~0~1  YMax=160~90000~1100~4
  Power : Subsystem
  Relational Operator : RelationalOperator  Operator===  ZeroCross=off  InputSameDT=on
  Selector : Selector  Elements=2  InputPortWidth=3
  Suction : Subsystem  TreatAsAtomicUnit=on
  Sum : Sum  Inputs=|-+  SaturateOnIntegerOverflow=on  InputSameDT=on
  Sum2 : Sum  Inputs=|++  SaturateOnIntegerOverflow=on  InputSameDT=on
  Sum3 : Sum  Inputs=|+-  SaturateOnIntegerOverflow=on  InputSameDT=on
  Force : Outport
  wires:
  Sum2/1 -> Piston2 Thermodynamics/4, Multiport Switch/1, Relational Operator/1
  [Sequence] -> Math Function/1
  Advance/1 -> Sum2/2
  Math Function/1 -> Sum2/1
  Constant3/1 -> Math Function/2
  PistonPos/1 -> Selector/1
  Selector/1 -> Sum/1
  Relational Operator/1 -> Power/3(Spark)
  Area/1 -> Force/1
  Sum/1 -> CylnVol/1
  Constant/1 -> Relational Operator/2
  Demux1/1 -> Piston2 Thermodynamics/1
  Compression/1(T_P) -> Multiport Switch/4, Power/1(Temperature_Pressure)
  CylnVol/1 -> Piston2 Thermodynamics/3, Power/2(Volume), Compression/1(Volume)
  Constant1/1 -> Sum/2
  Fuel/1 -> Power/4(Fuel)
  Power/1(T_P) -> Multiport Switch/5
  Demux1/2 -> Piston2 Thermodynamics/2, Sum3/1
  Sum3/1 -> Area/1
  Pa/1 -> Sum3/2
  Multiport Switch/1 -> Demux1/1
  Exhaust/1(T_P) -> Multiport Switch/2
  Suction/1(T_P) -> Multiport Switch/3

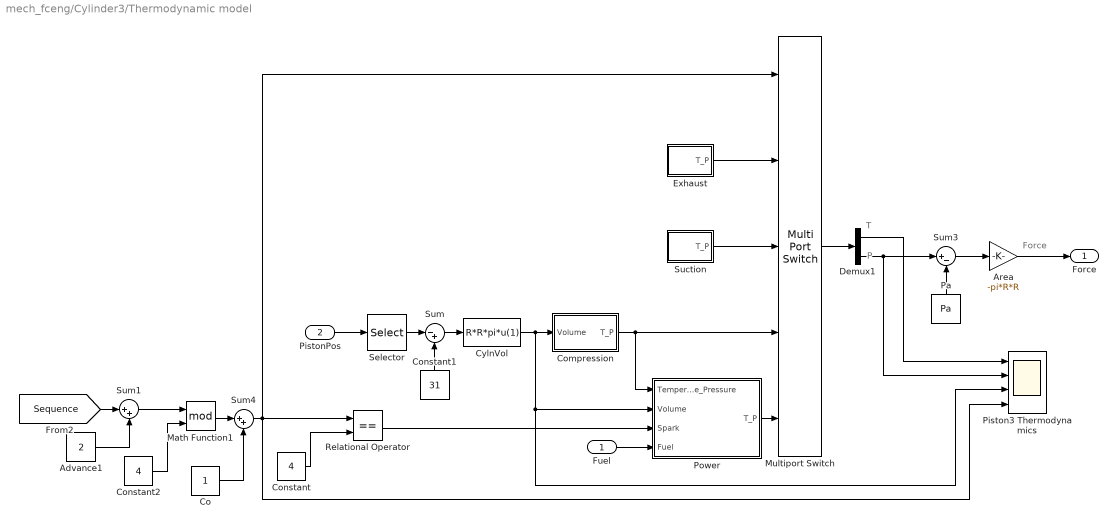
== system mech_fceng/Cylinder3/Thermodynamic model ==
  note: Force
  note: P
  note: T
  Fuel : Inport  Port=1  LatchInput=off
  PistonPos : Inport  Port=2  LatchInput=off
  Advance1 : Constant  Value=2
  Area : Gain  Gain=-pi*R*R  SaturateOnIntegerOverflow=on
  Co : Constant
  Compression : Subsystem
  Constant : Constant  Value=4
  Constant1 : Constant  Orientation=up  Value=31
  Constant2 : Constant  Value=4
  CylnVol : Fcn  Expr=R*R*pi*u(1)
  Demux1 : Demux  Outputs=2
  Exhaust : Subsystem  TreatAsAtomicUnit=on
  Math Function1 : Math  Operator=mod  SaturateOnIntegerOverflow=on
  Multiport Switch : MultiPortSwitch  InputSameDT=on
  Pa : Constant  Orientation=up  Value=Pa
  Piston3 Thermodynamics : Scope  NumInputPorts=4
      settings: TimeRange=20  YMin=25~0~0~1  YMax=350~200000~1100~4
  Power : Subsystem
  Relational Operator : RelationalOperator  Operator===  ZeroCross=off  InputSameDT=on
  Selector : Selector  Elements=2  InputPortWidth=3
  Suction : Subsystem  TreatAsAtomicUnit=on
  Sum : Sum  Inputs=|-+  SaturateOnIntegerOverflow=on  InputSameDT=on
  Sum1 : Sum  Inputs=|++  SaturateOnIntegerOverflow=on  InputSameDT=on
  Sum3 : Sum  Inputs=|+-  SaturateOnIntegerOverflow=on  InputSameDT=on
  Sum4 : Sum  Inputs=|++  SaturateOnIntegerOverflow=on  InputSameDT=on
  Force : Outport
  wires:
  Advance1/1 -> Sum1/2
  [Sequence] -> Sum1/1
  Sum1/1 -> Math Function1/1
  Co/1 -> Sum4/2
  Math Function1/1 -> Sum4/1
  Constant2/1 -> Math Function1/2
  Sum4/1 -> Piston3 Thermodynamics/4, Multiport Switch/1, Relational Operator/1
  PistonPos/1 -> Selector/1
  Selector/1 -> Sum/1
  Relational Operator/1 -> Power/3(Spark)
  Area/1 -> Force/1
  Sum/1 -> CylnVol/1
  Constant/1 -> Relational Operator/2
  Demux1/1 -> Piston3 Thermodynamics/1
  Compression/1(T_P) -> Multiport Switch/4, Power/1(Temperature_Pressure)
  CylnVol/1 -> Piston3 Thermodynamics/3, Power/2(Volume), Compression/1(Volume)
  Constant1/1 -> Sum/2
  Fuel/1 -> Power/4(Fuel)
  Power/1(T_P) -> Multiport Switch/5
  Demux1/2 -> Piston3 Thermodynamics/2, Sum3/1
  Sum3/1 -> Area/1
  Pa/1 -> Sum3/2
  Multiport Switch/1 -> Demux1/1
  Exhaust/1(T_P) -> Multiport Switch/2
  Suction/1(T_P) -> Multiport Switch/3

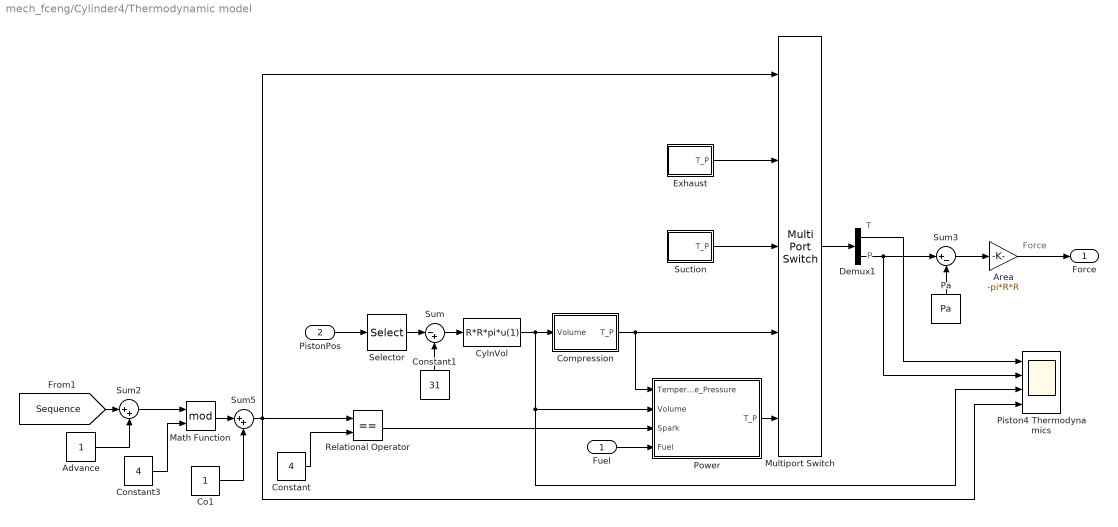
== system mech_fceng/Cylinder4/Thermodynamic model ==
  note: T
  note: P
  note: Force
  Fuel : Inport  Port=1  LatchInput=off
  PistonPos : Inport  Port=2  LatchInput=off
  Advance : Constant
  Area : Gain  Gain=-pi*R*R  SaturateOnIntegerOverflow=on
  Co1 : Constant
  Compression : Subsystem
  Constant : Constant  Value=4
  Constant1 : Constant  Orientation=up  Value=31
  Constant3 : Constant  Value=4
  CylnVol : Fcn  Expr=R*R*pi*u(1)
  Demux1 : Demux  Outputs=2
  Exhaust : Subsystem  TreatAsAtomicUnit=on
  Math Function : Math  Operator=mod  SaturateOnIntegerOverflow=on
  Multiport Switch : MultiPortSwitch  InputSameDT=on
  Pa : Constant  Orientation=up  Value=Pa
  Piston4 Thermodynamics : Scope  NumInputPorts=4
      settings: YMin=0~0~0~1  YMax=4500~2.5e+006~1100~4
  Power : Subsystem
  Relational Operator : RelationalOperator  Operator===  ZeroCross=off  InputSameDT=on
  Selector : Selector  Elements=2  InputPortWidth=3
  Suction : Subsystem  TreatAsAtomicUnit=on
  Sum : Sum  Inputs=|-+  SaturateOnIntegerOverflow=on  InputSameDT=on
  Sum2 : Sum  Inputs=|++  SaturateOnIntegerOverflow=on  InputSameDT=on
  Sum3 : Sum  Inputs=|+-  SaturateOnIntegerOverflow=on  InputSameDT=on
  Sum5 : Sum  Inputs=|++  SaturateOnIntegerOverflow=on  InputSameDT=on
  Force : Outport
  wires:
  Advance/1 -> Sum2/2
  [Sequence] -> Sum2/1
  Sum2/1 -> Math Function/1
  Co1/1 -> Sum5/2
  Math Function/1 -> Sum5/1
  Constant3/1 -> Math Function/2
  Suction/1(T_P) -> Multiport Switch/3
  Exhaust/1(T_P) -> Multiport Switch/2
  Multiport Switch/1 -> Demux1/1
  Pa/1 -> Sum3/2
  Sum3/1 -> Area/1
  Demux1/2 -> Sum3/1, Piston4 Thermodynamics/2
  Power/1(T_P) -> Multiport Switch/5
  Fuel/1 -> Power/4(Fuel)
  Constant1/1 -> Sum/2
  CylnVol/1 -> Compression/1(Volume), Power/2(Volume), Piston4 Thermodynamics/3
  Compression/1(T_P) -> Power/1(Temperature_Pressure), Multiport Switch/4
  Demux1/1 -> Piston4 Thermodynamics/1
  Constant/1 -> Relational Operator/2
  Sum/1 -> CylnVol/1
  Area/1 -> Force/1
  Relational Operator/1 -> Power/3(Spark)
  Selector/1 -> Sum/1
  PistonPos/1 -> Selector/1
  Sum5/1 -> Piston4 Thermodynamics/4, Relational Operator/1, Multiport Switch/1

== system mech_fceng/Engine Block/Engine Timer ==
  Angle : Inport  Orientation=left  Port=1  LatchInput=off
  Constant : Constant  Orientation=left  Value=pi/4
  Hit  Crossing2 : HitCross  Orientation=left  ZeroCross=off
  Ignition Control : Stateflow chart  Orientation=left  TreatAsAtomicUnit=on
  Sum : Sum  Orientation=left  Inputs=++|  SaturateOnIntegerOverflow=on  InputSameDT=on
  Trigonometric Function : Trigonometry  Orientation=left  Operator=cos
  tag scope: Sequence=global
  wires:
  Ignition Control/1(Sequence) -> [Sequence]
  Hit  Crossing2/1 -> Ignition Control/Trigger
  Trigonometric Function/1 -> Hit  Crossing2/1
  Sum/1 -> Ignition Control/1(CrankAngle), Trigonometric Function/1
  Constant/1 -> Sum/1
  Angle/1 -> Sum/2

== system mech_fceng/Engine Block/Friction ==
  Angle : Inport  Orientation=left  Port=1  LatchInput=off
  Rate : Inport  Orientation=left  Port=2  LatchInput=off
  Fcn : Fcn  Orientation=left  Expr=u < 0
  Gain : Gain  Orientation=left  Gain=1000  SaturateOnIntegerOverflow=on
  Gain1 : Gain  Orientation=left  Gain=-200  SaturateOnIntegerOverflow=on
  S-R Flip-Flop : simulink_extras/Flip Flops/S-R Flip-Flop  Orientation=left  initial_condition=0
  Sum1 : Sum  Orientation=left  Inputs=++|  SaturateOnIntegerOverflow=on  InputSameDT=on
  Torque : Outport  Orientation=left
  tag scope: CrankSR=global
  wires:
  Sum1/1 -> Torque/1
  Angle/1 -> [CrankSR], Fcn/1
  Rate/1 -> Gain1/1
  Gain1/1 -> Sum1/1
  Gain/1 -> Sum1/2
  S-R Flip-Flop/2 -> Gain/1
  Fcn/1 -> S-R Flip-Flop/1

== system mech_fceng/Cylinder1/Thermodynamic model/Compression ==
  note: Compression
  note: P
  note: T
  Volume : Inport  Port=1  LatchInput=off
  Mux : Mux  Inputs=2
  P : Fcn  Expr=Pa*(Vo/u(1))^G
  T : Fcn  Expr=Ta*(Vo/u(1))^(G-1)
  T_P : Outport
  wires:
  Volume/1 -> P/1, T/1
  Mux/1 -> T_P/1
  P/1 -> Mux/2
  T/1 -> Mux/1

== system mech_fceng/Cylinder1/Thermodynamic model/Exhaust ==
  note: Exhaust
  Mux : Mux  Inputs=2
  Pa : Constant  Value=Pa
  Ta : Constant  Value=Ta
  T_P : Outport
  wires:
  Mux/1 -> T_P/1
  Ta/1 -> Mux/1
  Pa/1 -> Mux/2

== system mech_fceng/Cylinder1/Thermodynamic model/Power ==
  Temperature_Pressure : Inport  Port=1  LatchInput=off
  Volume : Inport  Port=2  LatchInput=off
  Spark : Inport  Port=3  LatchInput=off
  Fuel : Inport  Port=4  LatchInput=off
  Combustion : Subsystem  TreatAsAtomicUnit=on
  Demux1 : Demux  Outputs=2
  IC : InitialCondition  Value=[Ta;Pa]
  IdealExpansion : Subsystem  TreatAsAtomicUnit=on
  Mux : Mux  Inputs=2
  T_P : Outport
  wires:
  Combustion/3(VolumeAfterCombustion) -> IdealExpansion/3(VolumeAfterCombustion)
  Combustion/1(TemperatureAfterCombustion) -> IdealExpansion/1(TemperatureAfterCombustion)
  IC/1 -> Demux1/1
  IdealExpansion/2(FPressure) -> Mux/2
  IdealExpansion/1(FTemperature) -> Mux/1
  Volume/1 -> Combustion/4(VolumeBeforeCombustion), IdealExpansion/4(IVolume)
  Combustion/2(PressureAfterCombustion) -> IdealExpansion/2(PressureAfterCombustion)
  Demux1/2 -> Combustion/2(PressureBeforeCombustion)
  Demux1/1 -> Combustion/1(TemperatureBeforeCombustion)
  Temperature_Pressure/1 -> IC/1
  Spark/1 -> Combustion/Trigger
  Fuel/1 -> Combustion/3(Fuel)
  Mux/1 -> T_P/1

== system mech_fceng/Cylinder1/Thermodynamic model/Suction ==
  note: Suction
  Mux : Mux  Inputs=2
  Pa : Constant  Value=Pa
  Ta : Constant  Value=Ta
  T_P : Outport
  wires:
  Pa/1 -> Mux/2
  Ta/1 -> Mux/1
  Mux/1 -> T_P/1

== system mech_fceng/Cylinder2/Thermodynamic model/Compression ==
  note: Compression
  note: P
  note: T
  Volume : Inport  Port=1  LatchInput=off
  Mux : Mux  Inputs=2
  P : Fcn  Expr=Pa*(Vo/u(1))^G
  T : Fcn  Expr=Ta*(Vo/u(1))^(G-1)
  T_P : Outport
  wires:
  Volume/1 -> P/1, T/1
  Mux/1 -> T_P/1
  P/1 -> Mux/2
  T/1 -> Mux/1

== system mech_fceng/Cylinder2/Thermodynamic model/Exhaust ==
  note: Exhaust
  Mux : Mux  Inputs=2
  Pa : Constant  Value=Pa
  Ta : Constant  Value=Ta
  T_P : Outport
  wires:
  Mux/1 -> T_P/1
  Ta/1 -> Mux/1
  Pa/1 -> Mux/2

== system mech_fceng/Cylinder2/Thermodynamic model/Power ==
  Temperature_Pressure : Inport  Port=1  LatchInput=off
  Volume : Inport  Port=2  LatchInput=off
  Spark : Inport  Port=3  LatchInput=off
  Fuel : Inport  Port=4  LatchInput=off
  Combustion : Subsystem  TreatAsAtomicUnit=on
  Demux1 : Demux  Outputs=2
  IC : InitialCondition  Value=[Ta;Pa]
  IdealExpansion : Subsystem  TreatAsAtomicUnit=on
  Mux : Mux  Inputs=2
  T_P : Outport
  wires:
  IC/1 -> Demux1/1
  IdealExpansion/2(FPressure) -> Mux/2
  IdealExpansion/1(FTemperature) -> Mux/1
  Volume/1 -> Combustion/4(VolumeBeforeCombustion), IdealExpansion/4(IVolume)
  Combustion/3(VolumeAfterCombustion) -> IdealExpansion/3(VolumeAfterCombustion)
  Combustion/2(PressureAfterCombustion) -> IdealExpansion/2(PressureAfterCombustion)
  Combustion/1(TemperatureAfterCombustion) -> IdealExpansion/1(TemperatureAfterCombustion)
  Demux1/2 -> Combustion/2(PressureBeforeCombustion)
  Demux1/1 -> Combustion/1(TemperatureBeforeCombustion)
  Temperature_Pressure/1 -> IC/1
  Spark/1 -> Combustion/Trigger
  Fuel/1 -> Combustion/3(Fuel)
  Mux/1 -> T_P/1

== system mech_fceng/Cylinder2/Thermodynamic model/Suction ==
  note: Suction
  Mux : Mux  Inputs=2
  Pa : Constant  Value=Pa
  Ta : Constant  Value=Ta
  T_P : Outport
  wires:
  Pa/1 -> Mux/2
  Ta/1 -> Mux/1
  Mux/1 -> T_P/1

== system mech_fceng/Cylinder3/Thermodynamic model/Compression ==
  note: Compression
  note: P
  note: T
  Volume : Inport  Port=1  LatchInput=off
  Mux : Mux  Inputs=2
  P : Fcn  Expr=Pa*(Vo/u(1))^G
  T : Fcn  Expr=Ta*(Vo/u(1))^(G-1)
  T_P : Outport
  wires:
  Volume/1 -> P/1, T/1
  Mux/1 -> T_P/1
  P/1 -> Mux/2
  T/1 -> Mux/1

== system mech_fceng/Cylinder3/Thermodynamic model/Exhaust ==
  note: Exhaust
  Mux : Mux  Inputs=2
  Pa : Constant  Value=Pa
  Ta : Constant  Value=Ta
  T_P : Outport
  wires:
  Mux/1 -> T_P/1
  Ta/1 -> Mux/1
  Pa/1 -> Mux/2

== system mech_fceng/Cylinder3/Thermodynamic model/Power ==
  Temperature_Pressure : Inport  Port=1  LatchInput=off
  Volume : Inport  Port=2  LatchInput=off
  Spark : Inport  Port=3  LatchInput=off
  Fuel : Inport  Port=4  LatchInput=off
  Combustion : Subsystem  TreatAsAtomicUnit=on
  Demux1 : Demux  Outputs=2
  IC : InitialCondition  Value=[Ta;Pa]
  IdealExpansion : Subsystem  TreatAsAtomicUnit=on
  Mux : Mux  Inputs=2
  T_P : Outport
  wires:
  IC/1 -> Demux1/1
  IdealExpansion/2(FPressure) -> Mux/2
  IdealExpansion/1(FTemperature) -> Mux/1
  Volume/1 -> Combustion/4(VolumeBeforeCombustion), IdealExpansion/4(IVolume)
  Combustion/3(VolumeAfterCombustion) -> IdealExpansion/3(VolumeAfterCombustion)
  Combustion/2(PressureAfterCombustion) -> IdealExpansion/2(PressureAfterCombustion)
  Combustion/1(TemperatureAfterCombustion) -> IdealExpansion/1(TemperatureAfterCombustion)
  Demux1/2 -> Combustion/2(PressureBeforeCombustion)
  Demux1/1 -> Combustion/1(TemperatureBeforeCombustion)
  Temperature_Pressure/1 -> IC/1
  Spark/1 -> Combustion/Trigger
  Fuel/1 -> Combustion/3(Fuel)
  Mux/1 -> T_P/1

== system mech_fceng/Cylinder3/Thermodynamic model/Suction ==
  note: Suction
  Mux : Mux  Inputs=2
  Pa : Constant  Value=Pa
  Ta : Constant  Value=Ta
  T_P : Outport
  wires:
  Pa/1 -> Mux/2
  Ta/1 -> Mux/1
  Mux/1 -> T_P/1

== system mech_fceng/Cylinder4/Thermodynamic model/Compression ==
  note: T
  note: P
  note: Compression
  Volume : Inport  Port=1  LatchInput=off
  Mux : Mux  Inputs=2
  P : Fcn  Expr=Pa*(Vo/u(1))^G
  T : Fcn  Expr=Ta*(Vo/u(1))^(G-1)
  T_P : Outport
  wires:
  T/1 -> Mux/1
  P/1 -> Mux/2
  Mux/1 -> T_P/1
  Volume/1 -> T/1, P/1
